simulink model "test_color_power_led_01"  (Simulink 8.8)
settings: Solver=FixedStepDiscrete  StartTime=0.0  StopTime=10.0  FixedStep=0.002  RelTol=1e-3  EnableMultiTasking=on
InitFcn:
  | px4_ap1_mdl_callback('check_model');
libraries: px4_ap1_color_power_led_lib x1, px4_ap1_px4setup_lib x1
settings Model: Creator=Privat  LastModifiedBy=Privat
settings OptimizationCC: ExpressionDepthLimit=2147483647  InitFltsAndDblsToZero=on  LifeSpan=1
settings DebuggingCC: SolverPrmCheckMsg=warning  InheritedTsInSrcMsg=none
settings HardwareCC: ProdLargestAtomicInteger=Long  ProdLargestAtomicFloat=Float  ProdEndianess=LittleEndian  ProdHWDeviceType=ARM Compatible->ARM 7
settings SFSimCC: SimParseCustomCode=off
settings RTWCC: SystemTargetFile=px4_ap1.tlc  GenCodeOnly=on  GenerateMakefile=off
settings CodeAppCC: IgnoreCustomStorageClasses=off  CustomSymbolStrType=$N$R$M  InternalIdentifier=Classic
settings STFCustomTargetCC: TargetLangStandard=C99 (ISO)  ModelReferenceCompliant=off  IncludeMdlTerminateFcn=off  CombineOutputUpdateFcns=on  ERTCustomFileBanners=on  SupportContinuousTime=off  SupportNonInlinedSFcns=off  RemoveResetFunc=on  MATLABClassNameForMDSCustomization=Simulink.SoftwareTarget.ERTCustomization  CPPClassGenCompliant=on  GRTInterface=off  SystemTargetFile=px4_ap1.tlc
settings ERTTargetCC: TargetLangStandard=C99 (ISO)  MultiwordLength=2048  ModelReferenceCompliant=off  ParMdlRefBuildCompliant=off  CompOptLevelCompliant=off  ConcurrentExecutionCompliant=off  IncludeMdlTerminateFcn=off  ERTFirstTimeCompliant=off  ModelStepFunctionPrototypeControlCompliant=off  UseToolchainInfoCompliant=off  ExtModeMexFile=noextcomm  ERTSrcFileBannerTemplate=px4_ap1_code_template.cgt  ERTHdrFileBannerTemplate=px4_ap1_code_template.cgt  ERTDataSrcFileTemplate=px4_ap1_code_template.cgt  ERTDataHdrFileTemplate=px4_ap1_code_template.cgt  ERTCustomFileTemplate=px4_ap1_main.tlc  ConvertIfToSwitch=off  SuppressUnreachableDefaultCases=off

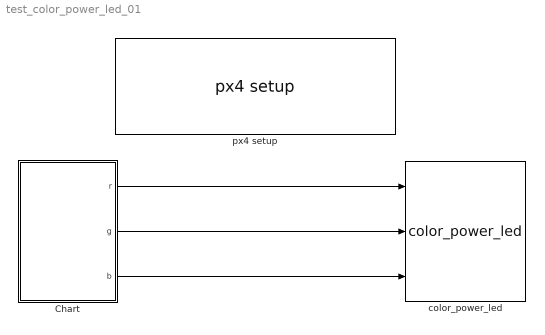
== system test_color_power_led_01 ==
  Chart : Stateflow chart  TreatAsAtomicUnit=on
  color_power_led : px4_ap1_color_power_led_lib/color_power_led
  px4 setup : px4_ap1_px4setup_lib/px4 setup  SampleTimeValue=0.002  cbBuild=on  cbUpload=off  cbPort=COM3  cpuLoad=off  debugmode=on
  wires:
  Chart/1(r) -> color_power_led/1
  Chart/2(g) -> color_power_led/2
  Chart/3(b) -> color_power_led/3

== stateflow chart Chart ==
  state RED
    en:
    r = 16;
    g = 0;
    b = 0;
  state BLUE
    en:
    r = 0;
    g = 0;
    b = 16;
  state GREEN
    en:
    r = 0;
    g = 17;
    b = 0;
  (default) -> RED
  RED -> BLUE : after(1,sec)
  GREEN -> RED : after(1,sec)
  BLUE -> GREEN : after(1,sec)
  data: r output uint32; g output uint32; b output uint32
